simulink model "thermal_system"  (R2023a)
settings: Solver=VariableStepAuto  StartTime=0.0  StopTime=1000  RelTol=1e-3
settings Model: Creator=Lucca  LastModifiedBy=Lucca

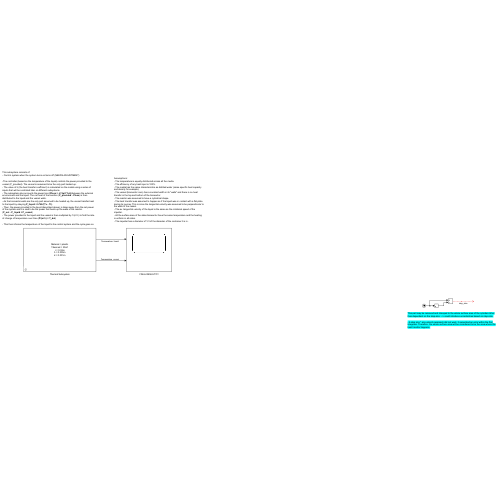
[thumbnail: Simulink's stored preview of the top-level diagram]
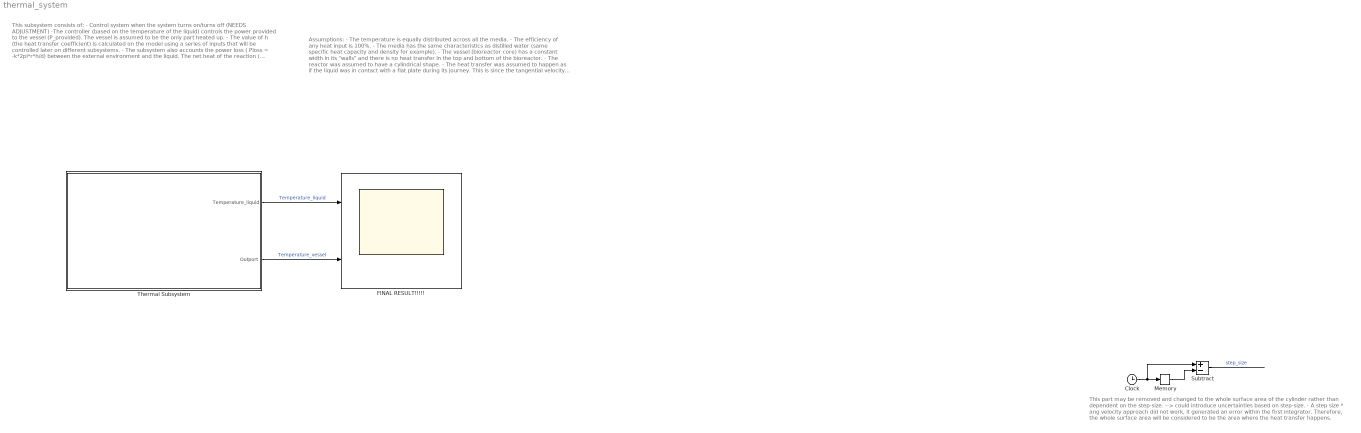
== system thermal_system ==
  note: This subsystem consists of:
      | - Control system when the system turns on/turns off (NEEDS ADJUSTMENT)
      |
      | -The controller (based on the temperature of the liquid) controls the power provided to the vessel (P_provided). The vessel is assumed to be the only part heated up.
      | - The value of h (the heat transfer coefficient) is calculated on the model using a series of inputs that will be controlled later on different subsystems.
      | - The subsystem also accounts the power loss ( Ploss = -k*2pi*r*h/d) between the external environment and the liquid. The net heat of the reaction ( P_provided - Ploss ) is then distributed to the liquid and the vessel walls.
      | - As the bioreactor walls are the only part assumed to be heated up, the vessel transfer heat to the liquid by obeying P_liquid = h*SA*(Tv - Tl).
      | - Then, the power provided to the liquid (described above) is taken away from the net power of the system and it is said to be the power that heats up the walls of the reactor.
      | ( P_net - P_liquid = P_vessel )
      | - The power provided to the liquid and the vessel is then multiplied by 1/(m*c) to find the rate of change of temperature over time ( P/(m*c) = T_dot )
      |
      | - This then informs the temperature of the liquid to the control system and the cycle goes on.
  note: This part may be removed and changed to the whole surface area of the cylinder rather than dependent on the step-size. --> could introduce uncertainties based on step-size.
      |
      | - A step size * ang velocity approach did not work, it generated an error within the first integrator. Therefore, the whole surface area will be considered to be the area where the heat transfer happens.
  note: Assumptions:
      | - The temperature is equally distributed across all the media.
      | - The efficiency of any heat input is 100%.
      | - The media has the same characteristics as distilled water (same specific heat capacity and density for example).
      | - The vessel (bioreactor core) has a constant width in its "walls" and there is no heat transfer in the top and bottom of the bioreactor.
      | - The reactor was assumed to have a cylindrical shape.
      | - The heat transfer was assumed to happen as if the liquid was in contact with a flat plate during its journey. This is since the tangential velocity was assumed to be perpendicular to the walls of the vessel.
      | - The av. tangential velocity of the liquid is the same as the rotational speed of the impeller.
      | - All the surface area of the sides bioreactor have the same temperature and the heating is uniform in all sides.
      | - The impeller has a diameter of 1/3 of the diameter of the container it is in.
  Clock : Clock
  FINAL RESULT!!!!! : Scope  NumInputPorts=2
  Memory : Memory
  Subtract : Sum  Inputs=+-
  Thermal Subsystem : Subsystem  mask{material=plastic, r=0.02, h=0.005, d=0.001, ml=0.25, cl=4180, Tenv=25, Tf=30, mv=2, Pheat=100}
      mask prompts: material "Material of the walls"; r "r - radius of vessel (m)"; h "h - height of vessel (m)"; d "d - width of the vessel (m)"; ml "ml - mass of liquid (kg)"; cl "cl - specific heat of liquid (J/kg*K)"; Tenv "Tenv -  Ambient temperature (Celsiums)"; Tf "Tf - Desired final temperature (Celsiums)"; mv "mv - mass of vessel (kg)"; Pheat "Pheat - power of heating element (W)"
      mask init:
      | str01 = "Material = " + material;
      | str0 = "Tdesired = " + Tf + "oC";
      | str1 = "r = " + r + "m";
      | str2 = "h = " + h + "m";
      | str3 = "d = " + d + "m";
      | label = [str01; str0; str1; str2; str3];
      | 
      | switch material
      |     case 'plastic'
      |         cv = 1670;
      |         k = 0.3;
      |     case 'aluminium'
      |         cv = 897;
      |         k = 237;
      |     case 'glass'
      |         cv = 840;
      |         k = 1;
      |     case 'new material (change in code)'
      |         cv = 1;
      |         k = 1;
      |         
      |         
      |         
      | end
      mask TypeOptions material: plastic | aluminium | glass | new material (change in code)
      mask Display: disp(label);
  wires:
  Thermal Subsystem/1(Temperature_liquid) -> FINAL RESULT!!!!!/1  "Temperature_liquid"
  Clock/1 -> Subtract/1, Memory/1
  Memory/1 -> Subtract/2
  Subtract/1 -> ?  "step_size"
  Thermal Subsystem/2(Outport) -> FINAL RESULT!!!!!/2  "Temperature_vessel"

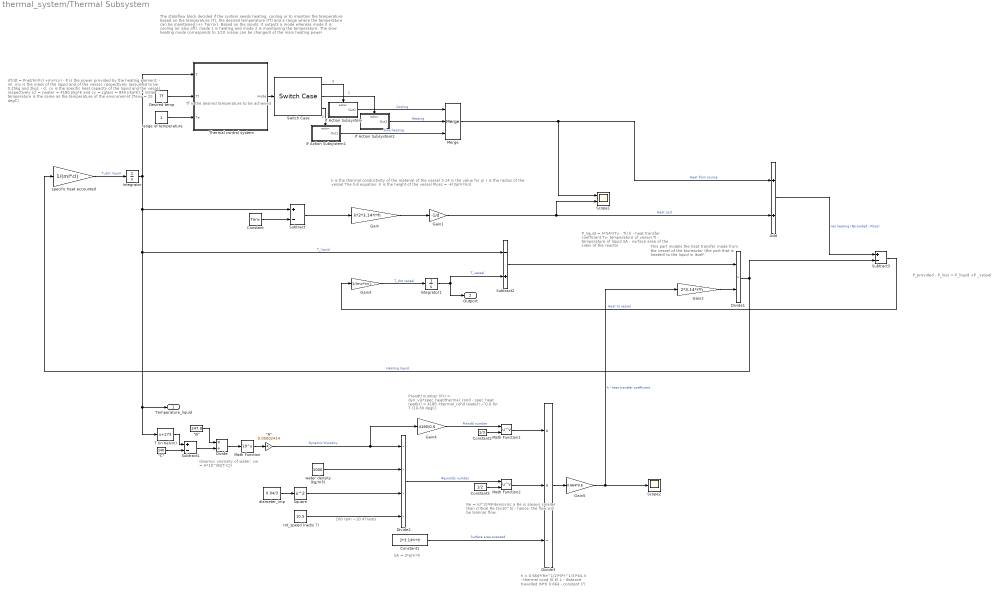
== system thermal_system/Thermal Subsystem ==
  note: This part models the heat transfer made from the vessel of the bioreactor (the part that is heated) to the liquid in itself.
  note: P_liquid = h*SA*(Tv - Tl)
      |
      | h - heat transfer coefficient
      | Tv- temperature of vessel
      | Tl - temperature of liquid
      | SA - surface area of the sides of the reactor
  note: SA = 2*pi*r*h
  note: P_provided - P_loss = P_liquid +P _vessel
  note: dinamyc viscosity of water:
      | vw = A*10^(B/[T-C])
  note: The stateflow block decided if the system needs heating, cooling or to maintain the temperature based on the temperature (T), the desired temperature (Tf) and a range where the temperature can be maintained (+/- Terror).
      |
      | Based on the inputs, it outputs a mode whereas mode 0 is cooling (or also off), mode 1 is heating and mode 2 is maintaining the temperature.
      |
      | The slow heating mode corresponds to 1/10 (value can be changed) of the main heating power
  note: Tf is the desired temperature to be achieved
  note: dT/dt = Pnet/(ml*cl +mv*cv)
      |
      | - P is the power provided by the heating element;
      | - ml, mv is the mass of the liquid and of the vessel, respectively (assumed to be 0.25kg and 2kg);
      | - cl, cv is the specific heat capacity of the liquid and the vessel respectively (cl = cwater = 4180 J/kg*K and cv = cglass = 840 J/kg*K);
      | - initial temperature is the same as the temperature of the environemnt (Tenv = 25 degC)
  note: k is the thermal conductivity of the material of the vessel
      | 3.14 is the value for pi
      | r is the radius of the vessel The full equation:
      | h is the height of the vessel Ploss = -k*2pi*r*h/d
  note: Prandtl number (Pr) = dyn_vis*spec_heat/thermal_cond
      |
      | - spec_heat (water) = 4180
      | -thermal_cond (water) ~ 0.6 for T (10-30 degC)
  note: Re = (d^2)*N*dens/visc
      | a
      | Re is always smaller than critical Re (5x10^5)
      | - hence, the flow will be laminar flow.
  note: h = 0.664*(Re^1/2)*(Pr^1/3)*k/L
      | k - thermal cond (0.6)
      | L - distance travelled (N*t)
      | 0.664 - constant (?)
  note: 100 rpm ~10.47rad/s
  "\"A\"" : Gain  Gain=0.00002414
  "\"B\"" : Constant  Value=247.8
  "\"C\"" : Constant  Value=140
  Add : Sum
  Constant : Constant  Value=Tenv
  Constant1 : Constant  Value=2*3.14*r*h
  Constant2 : Constant  Value=1/3
  Constant3 : Constant  Value=1/2
  Desired temp : Constant  Value=Tf
  Divide : Product  Inputs=*/
  Divide1 : Product  Inputs=**
  Divide2 : Product  Inputs=/***
  Divide3 : Product  Inputs=**/
  Gain : Gain  Gain=k*2*3.14*r*h
  Gain1 : Gain  Gain=-1/d
  Gain2 : Gain  Gain=2*3.14*r*h
  Gain3 : Gain  Gain=1/(mv*cv)
  Gain4 : Gain  Gain=4180/0.6
  Gain5 : Gain  Gain=0.664*0.6
  If Action Subsystem : Subsystem  TreatAsAtomicUnit=on
  If Action Subsystem1 : Subsystem  TreatAsAtomicUnit=on
  If Action Subsystem2 : Subsystem  TreatAsAtomicUnit=on
  Integrator : Integrator  InitialCondition=Tenv
  Integrator1 : Integrator  InitialCondition=Tenv
  Math Function : Math  Operator=10^u
  Math Function1 : Math  Operator=pow
  Math Function2 : Math  Operator=pow
  Merge : Merge  Inputs=3
  Scope1 : Scope  NumInputPorts=2
  Scope2 : Scope
  Square : Math  Operator=square
  Subtract : Sum  Inputs=+-
  Subtract1 : Sum  Inputs=+-
  Subtract2 : Sum  Inputs=-+
  Subtract3 : Sum  Inputs=+-
  Switch Case : SwitchCase  CaseConditions={0,1,2}  ShowDefaultCase=off
  T (in Kelvin) : Bias  Bias=273  SaturateOnIntegerOverflow=off
  Thermal control system : Stateflow chart  TreatAsAtomicUnit=on
  diameter_imp : Constant  Value=0.04/3
  range of temperature : Constant
  rot_speed (rad/s ?) : Constant  Value=10.5
  specific heat accounted : Gain  Gain=1/(ml*cl)
  "water density (kg/m3) " : Constant  Value=1000
  Temperature_liquid : Outport
  Outport : Outport  Port=2
  wires:
  Switch Case/3 -> If Action Subsystem1/Action  "2"
  Thermal control system/1(mode) -> Switch Case/1
  Desired temp/1 -> Thermal control system/2(Tf)
  If Action Subsystem2/1(Out1) -> Merge/2  "Heating"
  specific heat accounted/1 -> Integrator/1  "T_dot liquid"
  Integrator/1 -> Temperature_liquid/1, T (in Kelvin)/1, Subtract2/1, Subtract/1, Thermal control system/1(T)  "T_liquid"
  Switch Case/2 -> If Action Subsystem2/Action  "1"
  If Action Subsystem/1(Out1) -> Merge/1  "Cooling"
  If Action Subsystem1/1(Out1) -> Merge/3  "Slow heating"
  Switch Case/1 -> If Action Subsystem/Action  "0"
  range of temperature/1 -> Thermal control system/3(Te)
  Merge/1 -> Add/1, Scope1/1  "Heat from source"
  Constant/1 -> Subtract/2
  Subtract/1 -> Gain/1
  Gain/1 -> Gain1/1
  Gain1/1 -> Scope1/2, Add/2  "Heat Lost"
  T (in Kelvin)/1 -> Subtract1/1
  "\"C\""/1 -> Subtract1/2
  Subtract1/1 -> Divide/2
  "\"B\""/1 -> Divide/1
  Divide/1 -> Math Function/1
  Math Function/1 -> "\"A\""/1
  Gain3/1 -> Integrator1/1  "T_dot vessel"
  Integrator1/1 -> Outport/1, Subtract2/2  "T_vessel"
  Subtract2/1 -> Divide1/1
  Gain2/1 -> Divide1/2
  Divide1/1 -> Subtract3/2, specific heat accounted/1  "Heating liquid"
  Add/1 -> Subtract3/1  "net heating (Pprovided - Ploss)"
  Subtract3/1 -> Gain3/1  "Heat to vessel"
  Constant1/1 -> Divide3/3  "Surface area exposed"
  Math Function2/1 -> Divide3/2
  Constant3/1 -> Math Function2/2
  diameter_imp/1 -> Square/1
  Gain4/1 -> Math Function1/1  "Prandtl number"
  Math Function1/1 -> Divide3/1
  Divide2/1 -> Math Function2/1  "Reynolds number"
  Divide3/1 -> Gain5/1
  "water density (kg/m3) "/1 -> Divide2/2
  Gain5/1 -> Scope2/1, Gain2/1  "h - heat transfer coefficient"
  Square/1 -> Divide2/3
  rot_speed (rad/s ?)/1 -> Divide2/4
  Constant2/1 -> Math Function1/2
  "\"A\""/1 -> Divide2/1, Gain4/1  "Dynamic Viscosity"

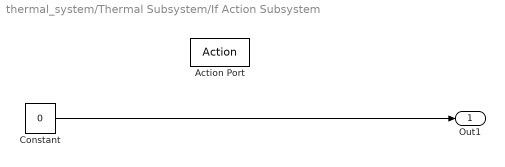
== system thermal_system/Thermal Subsystem/If Action Subsystem ==
  Action Port : ActionPort  ActionPortLabel=case [ 0 ]:
  Constant : Constant  Value=0
  Out1 : Outport
  wires:
  Constant/1 -> Out1/1

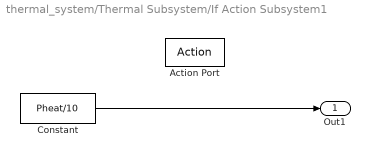
== system thermal_system/Thermal Subsystem/If Action Subsystem1 ==
  Action Port : ActionPort  ActionPortLabel=case [ 2 ]:
  Constant : Constant  Value=Pheat/10
  Out1 : Outport
  wires:
  Constant/1 -> Out1/1

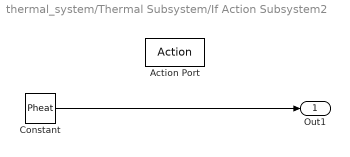
== system thermal_system/Thermal Subsystem/If Action Subsystem2 ==
  Action Port : ActionPort  ActionPortLabel=case [ 1 ]:
  Constant : Constant  Value=Pheat
  Out1 : Outport
  wires:
  Constant/1 -> Out1/1

== stateflow chart thermal_system/Thermal Subsystem/Thermal control system ==
  state Heating
    entry:
    mode = 1;
  state Cooling
    entry:
    mode = 0;
  state Slow_Heating
    entry:
    mode = 2;
  note: This part of the transition between cooling and slow heating can be observed to be changed (to save power, the slow heating part can be disabled after it reaches a certain temperature)
  Cooling -> Heating [order 1] : [T < (Tf-Te) ]
  Heating -> Cooling [order 2] : [T > (Tf+Te)]
  Cooling -> Slow_Heating [order 2] : [T < Tf]
  Slow_Heating -> Cooling [order 2] : [T > Tf]
  Heating -> Slow_Heating [order 1] : [T > (Tf-Te)]
  Slow_Heating -> Heating [order 1] : [T < (Tf-Te)]
  (default) -> Slow_Heating
  data: T input; Tf input; mode output; Te input
